simulink model "gui_experiment_supervisor"  (R2024b)
settings: Solver=FixedStepDiscrete  StartTime=0.0  StopTime=inf  FixedStep=Ts  RelTol=1e-3
model workspace (MAT data in the model file):
  Ts = Simulink.Parameter
  Ts.Value = 0.01
  Ts.Complexity = 'real'
  Ts.Dimensions = [1 1]
  Ts.DataType = 'auto'
  Ts.DocUnits = 's'
  board_ID = Simulink.Parameter
  board_ID.Value = 1
  board_ID.Complexity = 'real'
  board_ID.Dimensions = [1 1]
  board_ID.DataType = 'auto'
undefined symbols (not defined in the file): CAN_ANGLE_DEG2ICUB, CAN_ANGLE_ICUB2DEG, canChannel, ControlModes
libraries: canmsglib x12, canlib x4, simulink x1, dspsrcs4 x1, dspsigops x1, dspswit3 x1, sldrtlib x1
settings Model: DataDictionary=amcbldc.sldd  Creator=upattacini  LastModifiedBy=rpumpo
settings SolverCC: AlgebraicLoopSolver=TrustRegion  DecoupledContinuousIntegration=on  MinimalZcImpactIntegration=on
settings OptimizationCC: ReuseModelBlockBuffer=off  SimCompilerOptimization=on
settings DebuggingCC: ParameterPrecisionLossMsg=none  UnconnectedInputMsg=warning  UnconnectedOutputMsg=warning  UnconnectedLineMsg=warning  ArithmeticOperatorsInVariantConditions=warning
settings HardwareCC: ProdBitPerLong=64  ProdHWDeviceType=Intel->x86-64 (Linux 64)
settings ModelReferenceCC: EnableRefExpFcnMdlSchedulingChecks=on
settings SFSimCC: SimUseLocalCustomCode=off  CustomCodeUndefinedFunction=UseInterfaceOnly
settings RTWCC: Description=Simulink Desktop Real-Time  SystemTargetFile=sldrt.tlc  TemplateMakefile=sldrt.tmf  RTWUseLocalCustomCode=off  RTWCompilerOptimization=on  GPUComputeCapability=3.5  DLArmComputeVersion=19.05
settings CodeAppCC: MaxIdLength=95
settings SimulinkDesktopRealTimeCC: TargetLibSuffix=_sldrt.a  TargetPreCompLibLocation=C:\Program Files\MATLAB\R2024b\toolbox\sldrt\lib\win64  ParMdlRefBuildCompliant=on

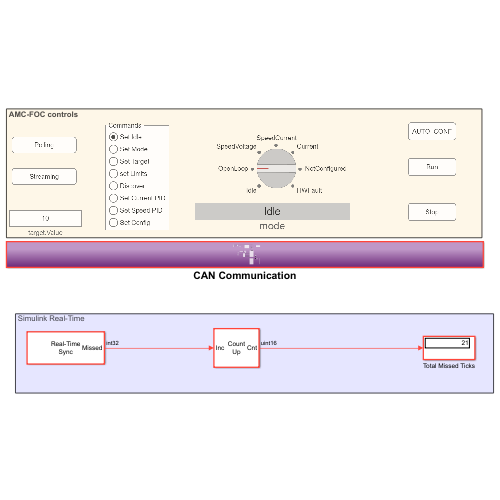
[thumbnail: Simulink's stored preview of the top-level diagram]
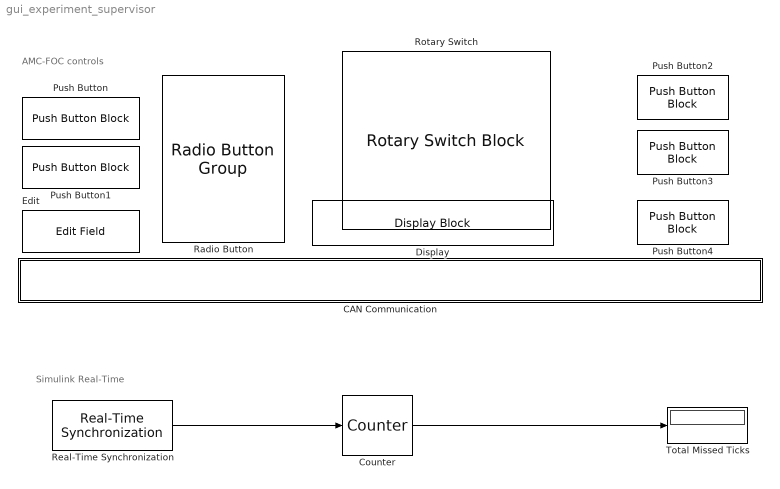
== system gui_experiment_supervisor ==
  note: AMC-FOC controls
  note: Simulink Real-Time
  CAN Communication : Subsystem
  Counter : dspswit3/Counter  Direction=Up  CountEvent=Rising edge  CounterSize=16 bits  MaxCount=10000  InitialCount=0  Output=Count  HitValue=32  ResetInput=off  SamplesPerFrame=1  Ts=1  CntDtype=uint16  HitDtype=Logical
  Display : DisplayBlock  LabelPosition=Bottom  Format=Integer  Transparency=1  FormatString=%s
  Edit : EditField  LabelPosition=Bottom  ShowInitialText=on  Alignment=Center
  Push Button : PushButtonBlock  ButtonText=Polling  OffValue=0.000000
  Push Button1 : PushButtonBlock  ButtonText=Streaming  ButtonType=Latch  OffValue=0.000000
  Push Button2 : PushButtonBlock  ButtonText=AUTO_CONF  OffValue=0.000000
  Push Button3 : PushButtonBlock  ButtonText=Run  OffValue=0.000000
  Push Button4 : PushButtonBlock  ButtonText=Stop  OffValue=0.000000
  Radio Button : RadioButtonGroup  LabelPosition=Hide  SelectedLabel=Set Idle  ButtonGroupName=Commands
      settings: Values={{'Set Idle', 'Set Mode', 'Set Target', 'set Limits', 'Discover', 'Set Current PID', 'Set Speed PID', 'Set Config'}, [1 2 3 4 5 6 7 8]}
  Real-Time Synchronization : sldrtlib/Real-Time Synchronization  SampleTime=Ts  MaxMissedTicks=inf  ShowMissedTicks=on  YieldWhenWaiting=off
  Rotary Switch : RotarySwitchBlock  LabelPosition=Hide  UseEnumeratedDataType=on  EnumeratedDataType=MCControlModes
      settings: Values={{'Idle', 'OpenLoop', 'SpeedVoltage', 'SpeedCurrent', 'Current', 'NotConfigured', 'HWFault'}, [0 80 10 11 6 176 160]}
  Total Missed Ticks : Display
      settings: Decimation=5
  wires:
  Counter/1 -> Total Missed Ticks/1
  Real-Time Synchronization/1 -> Counter/1

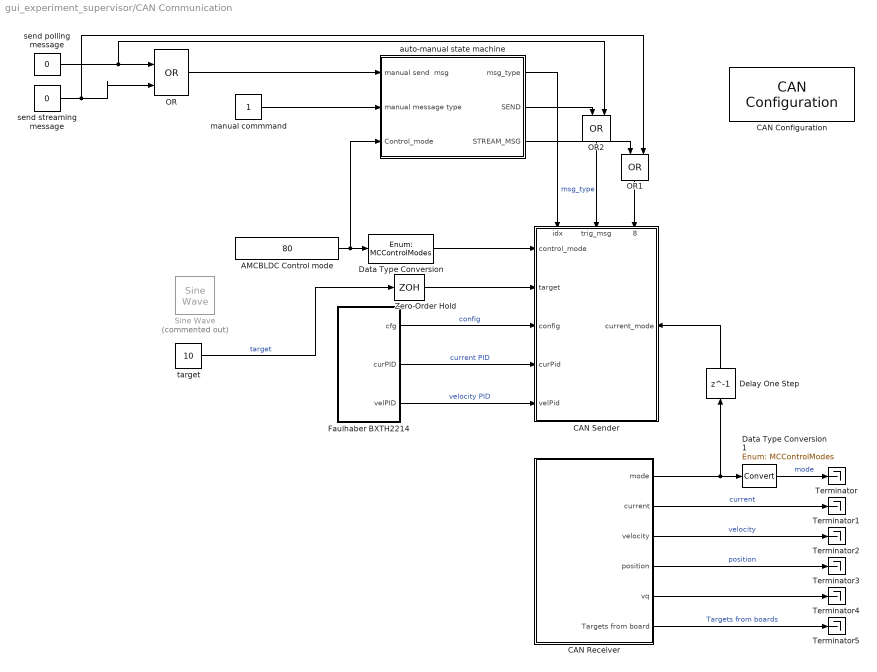
== system gui_experiment_supervisor/CAN Communication ==
  AMCBLDC Control mode : Constant  Value=80  OutDataTypeStr=int16  SampleTime=Ts
  CAN Configuration : canlib/CAN Configuration  BlockHandle=364.0001  Device=Vector VN1610 1 (Channel 1)  DeviceMenu=Vector VN1610 1 (Channel 1)  ObjConstructor=canChannel('Vector', 'VN1610 1', 1)  BusSpeed=1000000  EnableBitParameters=off  SJW=1  TSEG1=4  TSEG2=3  NSamples=1  AckMode=Normal
  CAN Receiver : Subsystem
  CAN Sender : Subsystem
      settings: PortSchema="{\"entries\":[{\"content\":{\"sides\":[{\"content\":{\"connectorIds\":[\"In1\",\"In2\",\"In3\",\"In4\",\"In5\"]},\"type\":\"ConnectorPlacement.EquallySpacedRectSide\",\"uuid\":\"bdd6ce9e-9b65-4aba-9b48-f09f8c1326bb\"},{\"content\":{\"connectorIds\":[\"In9\"],\"side\":\"RIGHT\"},\"type\":\"ConnectorPlacement.EquallySpacedRectSide\",\"uuid\":\"141c9ef5-f742-47fc-b635-015c7474b58f\"},{\"content\":{\"connectorIds\":[\"In6\",\"In7\",\"In8\"],\"side\":\"TOP\"},\"type\":\"ConnectorPlacement.EquallySpacedRectSide\",\"uuid\":\"624889ac-74c5-4b05-9d21-0587daea952f\"}]},\"type\":\"ConnectorPlacement.EquallySpacedConnector\",\"uuid\":\"a748afda-e52d-41b4-a312-ee668058905d\"}],\"packageUris\":[\"http://schema.mathworks.com/mf0/Connector/R2020b\"],\"version\":\"1.0\"}"
  Data Type Conversion : DataTypeConversion  OutDataTypeStr=Enum: MCControlModes  SaturateOnIntegerOverflow=off  RndMeth=Floor
  Data Type Conversion1 : DataTypeConversion  OutDataTypeStr=Enum: MCControlModes  SaturateOnIntegerOverflow=off  RndMeth=Floor
  Delay One Step : Delay  DelayLength=1
  Faulhaber BXTH2214 : Subsystem  TreatAsAtomicUnit=on  SystemSampleTime=Ts
  OR : Logic  Operator=OR  IconShape=distinctive  AllPortsSameDT=off  OutDataTypeStr=boolean
  OR1 : Logic  Operator=OR  IconShape=distinctive  AllPortsSameDT=off  OutDataTypeStr=boolean
  OR2 : Logic  Operator=OR  IconShape=distinctive  AllPortsSameDT=off  OutDataTypeStr=boolean
  Sine Wave : dspsrcs4/Sine Wave  Commented=on  Amplitude=1  Frequency=0.05  Phase=0  SampleMode=Discrete  OutComplex=Real  CompMethod=Trigonometric fcn  TableSize=Speed  SampleTime=1/50  SamplesPerFrame=1  ResetState=Restart at time zero  OutputFrames=off  dataType=double  wordLen=16  udDataType=sfix(16)  fracBitsMode=Best precision  numFracBits=15  OutDataTypeStr=double  LastOutDataTypeStr=double
  Terminator{,1..5} (6 alike) : Terminator
  Zero-Order Hold : ZeroOrderHold  SampleTime=Ts
  auto-manual state machine : Subsystem
  manual commmand : Constant  OutDataTypeStr=int16  SampleTime=Ts
  send polling message : Constant  Value=0  OutDataTypeStr=boolean  SampleTime=Ts
  send streaming message : Constant  Value=0  OutDataTypeStr=boolean  SampleTime=Ts
  target : Constant  Value=10  SampleTime=Ts
  wires:
  Faulhaber BXTH2214/2(curPID) -> CAN Sender/4(curPid)  "current PID"
  OR/1 -> auto-manual state machine/1(manual send  msg)
  Zero-Order Hold/1 -> CAN Sender/2(target)
  AMCBLDC Control mode/1 -> auto-manual state machine/3(Control_mode), Data Type Conversion/1
  CAN Receiver/3(velocity) -> Terminator2/1  "velocity"
  CAN Receiver/6(Targets from board) -> Terminator5/1  "Targets from boards"
  Data Type Conversion/1 -> CAN Sender/1(control_mode)
  Faulhaber BXTH2214/3(velPID) -> CAN Sender/5(velPid)  "velocity PID"
  CAN Receiver/5(vq) -> Terminator4/1
  CAN Receiver/4(position) -> Terminator3/1  "position"
  CAN Receiver/1(mode) -> Data Type Conversion1/1, Delay One Step/1
  manual commmand/1 -> auto-manual state machine/2(manual message type)
  auto-manual state machine/1(msg_type) -> CAN Sender/6(idx)  "msg_type"
  send streaming message/1 -> OR1/2, OR/2
  Data Type Conversion1/1 -> Terminator/1  "mode"
  send polling message/1 -> OR2/2, OR/1
  Delay One Step/1 -> CAN Sender/9(current_mode)
  Faulhaber BXTH2214/1(cfg) -> CAN Sender/3(config)  "config"
  target/1 -> Zero-Order Hold/1  "target"
  CAN Receiver/2(current) -> Terminator1/1  "current"
  auto-manual state machine/3(STREAM_MSG) -> OR1/1
  OR1/1 -> CAN Sender/8(trig_periodic)
  OR2/1 -> CAN Sender/7(trig_msg)
  auto-manual state machine/2(SEND) -> OR2/1

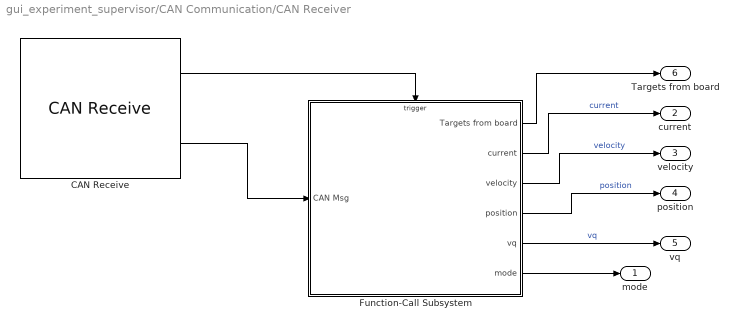
== system gui_experiment_supervisor/CAN Communication/CAN Receiver ==
  CAN Receive : canlib/CAN Receive  BlockHandle=372.0001  Device=Vector VN1610 1 (Channel 1)  DeviceMenu=Vector VN1610 1 (Channel 1)  ObjConstructor=canChannel('Vector', 'VN1610 1', 1)  EnableStandardIDsFilter=off  StdIDsCombo=Allow all  StandardIDs=0  EnableExtendedIDsFilter=off  ExtIDsCombo=Allow all  ExtendedIDs=0  SampleTime=Ts  MsgsPerTimestep=all  InternalFilterUpdateStatus=on  BusOutput=on
  Function-Call Subsystem : Subsystem  TreatAsAtomicUnit=on
  mode : Outport
  current : Outport  Port=2
  velocity : Outport  Port=3
  position : Outport  Port=4
  vq : Outport  Port=5
  Targets from board : Outport  Port=6
  wires:
  CAN Receive/1 -> Function-Call Subsystem/Trigger
  CAN Receive/2 -> Function-Call Subsystem/1(CAN Msg)
  Function-Call Subsystem/2(current) -> current/1  "current"
  Function-Call Subsystem/3(velocity) -> velocity/1  "velocity"
  Function-Call Subsystem/4(position) -> position/1  "position"
  Function-Call Subsystem/5(vq) -> vq/1  "vq"
  Function-Call Subsystem/1(Targets from board) -> Targets from board/1
  Function-Call Subsystem/6(mode) -> mode/1

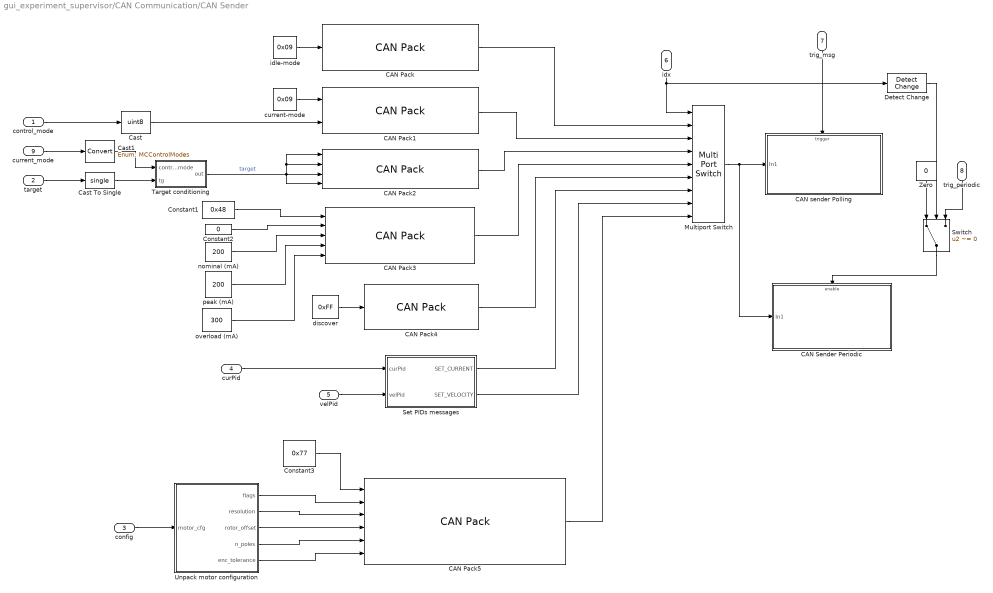
== system gui_experiment_supervisor/CAN Communication/CAN Sender ==
  control_mode : Inport
  target : Inport  Port=2
  config : Inport  Port=3
  curPid : Inport  Port=4
  velPid : Inport  Port=5
  idx : Inport  Port=6
  trig_msg : Inport  Port=7
  trig_periodic : Inport  Port=8
  current_mode : Inport  Port=9
  CAN Pack : canmsglib/CAN Pack  MsgList=(none)  MsgName=CAN Idle  MsgIDType=Standard (11-bit identifier)  MsgIdentifier=board_ID  CANIDInput=off  MsgLength=2  Remote=off  ApplyMinMax=off  BusOutput=on  SignalInfo={ 'Idle', '0', '16', 'LE', 'unsigned', 'Standard', '0', '1', '0', '-Inf', 'Inf' }
      settings: DataFormat=manually specified signals
  CAN Pack1 : canmsglib/CAN Pack  MsgList=(none)  MsgName=SET Control Mode  MsgIDType=Standard (11-bit identifier)  MsgIdentifier=board_ID  CANIDInput=off  MsgLength=2  Remote=off  ApplyMinMax=off  BusOutput=on  SignalInfo={ 'CMD', '0', '8', 'LE', 'unsigned', 'Standard', '0', '1', '0', '-Inf', 'Inf'; 'CTRL', '8', '8', 'LE', 'signed', 'Standard', '0', '1', '0', '-Inf', 'Inf' }
      settings: DataFormat=manually specified signals
  CAN Pack2 : canmsglib/CAN Pack  MsgList=(none)  MsgName=CAN Target  MsgIDType=Standard (11-bit identifier)  MsgIdentifier=0x10F  CANIDInput=off  MsgLength=8  Remote=off  ApplyMinMax=off  BusOutput=on  SignalInfo={ 'Target 1', '0', '16', 'LE', 'signed', 'Standard', '0', '1', '0', '-Inf', 'Inf'; 'Target 2', '16', '16', 'LE', 'signed', 'Standard', '0', '1', '0', '-Inf', 'Inf'; 'Target 3', '32', '16', 'LE', 'signed', 'Standard', '0', '1', '0', '-Inf', 'Inf'; 'Target 4', '48', '16', 'LE', 'signed', 'Standard', '0', '1', '0', '-Inf', 'Inf' }
      settings: DataFormat=manually specified signals
  CAN Pack3 : canmsglib/CAN Pack  MsgList=(none)  MsgName=CAN Limits  MsgIDType=Standard (11-bit identifier)  MsgIdentifier=board_ID  CANIDInput=off  MsgLength=8  Remote=off  ApplyMinMax=off  BusOutput=on  SignalInfo={ 'CMD', '0', '8', 'LE', 'unsigned', 'Standard', '0', '1', '0', '-Inf', 'Inf'; 'X', '8', '8', 'LE', 'unsigned', 'Standard', '0', '1', '0', '-Inf', 'Inf'; 'NOMINAL', '16', '16', 'LE', 'unsigned', 'Standard', '0', '1', '0', '-Inf', 'Inf'; 'PEAK', '32', '16', 'LE', 'unsigned', 'Standard', '0', '1', '0', '-Inf', 'Inf'; 'OVERLOAD', '48', '16', 'LE', 'unsigned', 'Standard', '0', '1', '0', '-Inf', 'Inf' }
      settings: DataFormat=manually specified signals
  CAN Pack4 : canmsglib/CAN Pack  MsgList=(none)  MsgName=DISCOVER  MsgIDType=Standard (11-bit identifier)  MsgIdentifier=0x70F  CANIDInput=off  MsgLength=1  Remote=off  ApplyMinMax=off  BusOutput=on  SignalInfo={}
      settings: DataFormat=raw data
  CAN Pack5 : canmsglib/CAN Pack  MsgList=(none)  MsgName=Set_Motor_Config  MsgIDType=Standard (11-bit identifier)  MsgIdentifier=board_ID  CANIDInput=off  MsgLength=8  Remote=off  ApplyMinMax=off  BusOutput=on  SignalInfo={ 'CMD', '0', '8', 'LE', 'unsigned', 'Standard', '0', '1', '0', '-Inf', 'Inf'; 'FLAGS', '8', '8', 'LE', 'unsigned', 'Standard', '0', '1', '0', '-Inf', 'Inf'; 'RES_ENCODER', '16', '16', 'LE', 'signed', 'Standard', '0', '1', '0', '-Inf', 'Inf'; 'OFFSET_ENCODER', '32', '16', 'LE', 'unsigned', 'Standard', '0', '1', '0', '-Inf', 'Inf'; 'N_POLES', '48', '8', 'LE', 'unsigned', 'Standard', '0', '1', '0', '-Inf', 'Inf'; 'ENCODER_TOLERANCE', '56', '8', 'LE', 'unsigned', 'Standard', '0', '1', '0', '-Inf', 'Inf' }
      settings: DataFormat=manually specified signals
  CAN Sender Periodic : Subsystem  TreatAsAtomicUnit=on
  CAN sender Polling : Subsystem
  Cast : DataTypeConversion  OutDataTypeStr=uint8  SaturateOnIntegerOverflow=off  RndMeth=Floor
  Cast To Single : DataTypeConversion  OutDataTypeStr=single  SaturateOnIntegerOverflow=off  RndMeth=Floor
  Cast1 : DataTypeConversion  OutDataTypeStr=Enum: MCControlModes  SaturateOnIntegerOverflow=off  RndMeth=Floor
  Constant1 : Constant  Value=0x48  OutDataTypeStr=Inherit: Inherit via back propagation
  Constant2 : Constant  Value=0  OutDataTypeStr=Inherit: Inherit via back propagation
  Constant3 : Constant  Value=0x77  OutDataTypeStr=Inherit: Inherit via back propagation
  Detect Change : simulink/Logic and Bit Operations/Detect Change  vinit=0  OutDataTypeStr=boolean
  Multiport Switch : MultiPortSwitch  Inputs=8  DiagnosticForDefault=Warning  SaturateOnIntegerOverflow=off  InputSameDT=off
  Set PIDs messages : Subsystem
  Switch : Switch  Criteria=u2 ~= 0  SaturateOnIntegerOverflow=off  InputSameDT=off
  Target conditioning : Subsystem
  Unpack motor configuration : MATLAB Function  TreatAsAtomicUnit=on
  Zero : Constant  Value=0  OutDataTypeStr=Inherit: Inherit via back propagation
  current-mode : Constant  Value=0x09  OutDataTypeStr=Inherit: Inherit via back propagation
  discover : Constant  Value=0xFF
  idle-mode : Constant  Value=0x09  OutDataTypeStr=Inherit: Inherit via back propagation
  nominal (mA) : Constant  Value=200  OutDataTypeStr=Inherit: Inherit via back propagation
  overload (mA) : Constant  Value=300  OutDataTypeStr=Inherit: Inherit via back propagation
  peak (mA) : Constant  Value=200  OutDataTypeStr=Inherit: Inherit via back propagation
  wires:
  CAN Pack/1 -> Multiport Switch/2
  CAN Pack1/1 -> Multiport Switch/3
  CAN Pack2/1 -> Multiport Switch/4
  idx/1 -> Multiport Switch/1, Detect Change/1
  idle-mode/1 -> CAN Pack/1
  current-mode/1 -> CAN Pack1/1
  Constant1/1 -> CAN Pack3/1
  CAN Pack3/1 -> Multiport Switch/5
  discover/1 -> CAN Pack4/1
  CAN Pack4/1 -> Multiport Switch/6
  trig_msg/1 -> CAN sender Polling/Trigger
  Constant2/1 -> CAN Pack3/2
  nominal (mA)/1 -> CAN Pack3/3
  peak (mA)/1 -> CAN Pack3/4
  overload (mA)/1 -> CAN Pack3/5
  trig_periodic/1 -> Switch/3
  Multiport Switch/1 -> CAN Sender Periodic/1(In1), CAN sender Polling/1(In1)
  control_mode/1 -> Cast/1
  Constant3/1 -> CAN Pack5/1
  Set PIDs messages/2(SET_VELOCITY) -> Multiport Switch/8
  Set PIDs messages/1(SET_CURRENT) -> Multiport Switch/7
  velPid/1 -> Set PIDs messages/2(velPid)
  CAN Pack5/1 -> Multiport Switch/9
  config/1 -> Unpack motor configuration/1(motor_cfg)
  curPid/1 -> Set PIDs messages/1(curPid)
  Unpack motor configuration/1(flags) -> CAN Pack5/2
  Unpack motor configuration/2(resolution) -> CAN Pack5/3
  Unpack motor configuration/3(rotor_offset) -> CAN Pack5/4
  Unpack motor configuration/4(n_poles) -> CAN Pack5/5
  Unpack motor configuration/5(enc_tolerance) -> CAN Pack5/6
  target/1 -> Cast To Single/1
  Target conditioning/1(out) -> CAN Pack2/4, CAN Pack2/1, CAN Pack2/2, CAN Pack2/3  "target"
  Cast/1 -> CAN Pack1/2
  Cast1/1 -> Target conditioning/1(control_mode)
  current_mode/1 -> Cast1/1
  Detect Change/1 -> Switch/2
  Zero/1 -> Switch/1
  Switch/1 -> CAN Sender Periodic/Enable
  Cast To Single/1 -> Target conditioning/2(tg)

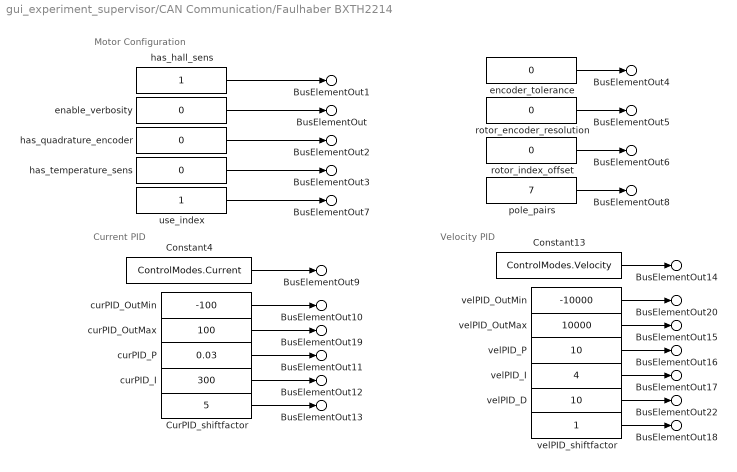
== system gui_experiment_supervisor/CAN Communication/Faulhaber BXTH2214 ==
  note: Motor Configuration
  note: Current PID
  note: Velocity PID
  Constant13 : Constant  Value=ControlModes.Velocity  OutDataTypeStr=Inherit: Inherit via back propagation
  Constant4 : Constant  Value=ControlModes.Current  OutDataTypeStr=Inherit: Inherit via back propagation
  CurPID_shiftfactor : Constant  Value=5  OutDataTypeStr=Inherit: Inherit via back propagation
  curPID_I : Constant  Value=300  OutDataTypeStr=Inherit: Inherit via back propagation
  curPID_OutMax : Constant  Value=100  OutDataTypeStr=Inherit: Inherit via back propagation
  curPID_OutMin : Constant  Value=-100  OutDataTypeStr=Inherit: Inherit via back propagation
  curPID_P : Constant  Value=0.03  OutDataTypeStr=Inherit: Inherit via back propagation
  enable_verbosity : Constant  Value=0  OutDataTypeStr=boolean
  encoder_tolerance : Constant  Value=0  OutDataTypeStr=Inherit: Inherit via back propagation
  has_hall_sens : Constant  OutDataTypeStr=boolean
  has_quadrature_encoder : Constant  Value=0  OutDataTypeStr=boolean
  has_temperature_sens : Constant  Value=0  OutDataTypeStr=boolean
  pole_pairs : Constant  Value=7  OutDataTypeStr=Inherit: Inherit via back propagation
  rotor_encoder_resolution : Constant  Value=0  OutDataTypeStr=Inherit: Inherit via back propagation
  rotor_index_offset : Constant  Value=0  OutDataTypeStr=Inherit: Inherit via back propagation
  use_index : Constant  OutDataTypeStr=boolean
  velPID_D : Constant  Value=10  OutDataTypeStr=Inherit: Inherit via back propagation
  velPID_I : Constant  Value=4  OutDataTypeStr=Inherit: Inherit via back propagation
  velPID_OutMax : Constant  Value=10000  OutDataTypeStr=Inherit: Inherit via back propagation
  "velPID_OutMin " : Constant  Value=-10000  OutDataTypeStr=Inherit: Inherit via back propagation
  velPID_P : Constant  Value=10  OutDataTypeStr=Inherit: Inherit via back propagation
  velPID_shiftfactor : Constant  OutDataTypeStr=Inherit: Inherit via back propagation
  BusElementOut : Outport  PortName=cfg  Element=enable_verbosity
  BusElementOut1 : Outport  PortName=cfg  Element=has_hall_sens
  BusElementOut2 : Outport  PortName=cfg  Element=has_quadrature_encoder
  BusElementOut3 : Outport  PortName=cfg  Element=has_temperature_sens
  BusElementOut4 : Outport  PortName=cfg  Element=encoder_tolerance
  BusElementOut8 : Outport  PortName=cfg  Element=pole_pairs
  BusElementOut5 : Outport  PortName=cfg  Element=rotor_encoder_resolution
  BusElementOut6 : Outport  PortName=cfg  Element=rotor_index_offset
  BusElementOut7 : Outport  PortName=cfg  Element=use_index
  BusElementOut9 : Outport  Port=2  PortName=curPID  Element=type
  BusElementOut19 : Outport  Port=2  PortName=curPID  Element=OutMax
  BusElementOut10 : Outport  Port=2  PortName=curPID  Element=OutMin
  BusElementOut11 : Outport  Port=2  PortName=curPID  Element=P
  BusElementOut12 : Outport  Port=2  PortName=curPID  Element=I
  BusElementOut13 : Outport  Port=2  PortName=curPID  Element=shift_factor
  BusElementOut14 : Outport  Port=3  PortName=velPID  Element=type
  BusElementOut15 : Outport  Port=3  PortName=velPID  Element=OutMax
  BusElementOut20 : Outport  Port=3  PortName=velPID  Element=OutMin
  BusElementOut16 : Outport  Port=3  PortName=velPID  Element=P
  BusElementOut17 : Outport  Port=3  PortName=velPID  Element=I
  BusElementOut22 : Outport  Port=3  PortName=velPID  Element=D
  BusElementOut18 : Outport  Port=3  PortName=velPID  Element=shift_factor
  wires:
  encoder_tolerance/1 -> BusElementOut4/1
  pole_pairs/1 -> BusElementOut8/1
  Constant4/1 -> BusElementOut9/1
  curPID_OutMin/1 -> BusElementOut10/1
  curPID_P/1 -> BusElementOut11/1
  curPID_OutMax/1 -> BusElementOut19/1
  curPID_I/1 -> BusElementOut12/1
  CurPID_shiftfactor/1 -> BusElementOut13/1
  velPID_I/1 -> BusElementOut17/1
  velPID_shiftfactor/1 -> BusElementOut18/1
  velPID_P/1 -> BusElementOut16/1
  Constant13/1 -> BusElementOut14/1
  rotor_encoder_resolution/1 -> BusElementOut5/1
  rotor_index_offset/1 -> BusElementOut6/1
  "velPID_OutMin "/1 -> BusElementOut20/1
  velPID_OutMax/1 -> BusElementOut15/1
  velPID_D/1 -> BusElementOut22/1
  enable_verbosity/1 -> BusElementOut/1
  has_quadrature_encoder/1 -> BusElementOut2/1
  has_temperature_sens/1 -> BusElementOut3/1
  use_index/1 -> BusElementOut7/1
  has_hall_sens/1 -> BusElementOut1/1

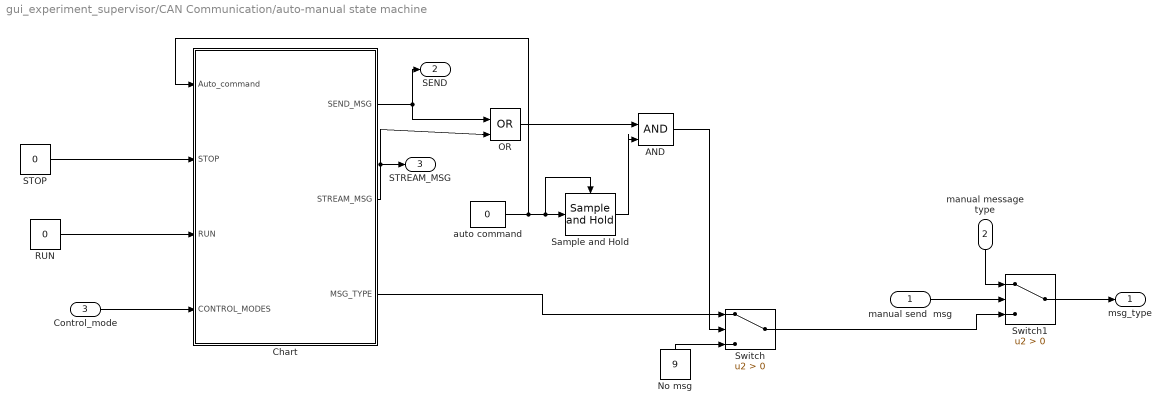
== system gui_experiment_supervisor/CAN Communication/auto-manual state machine ==
  manual send  msg : Inport
  manual message type : Inport  Port=2
  Control_mode : Inport  Port=3
  AND : Logic  IconShape=distinctive  AllPortsSameDT=off  OutDataTypeStr=boolean
  Chart : Stateflow chart  TreatAsAtomicUnit=on
      settings: PortSchema="{\"entries\":[{\"content\":{\"sides\":[{\"content\":{\"connectorIds\":[\"In1\",\"In3\",\"In2\",\"In4\"]},\"type\":\"ConnectorPlacement.EquallySpacedRectSide\",\"uuid\":\"3f3ecf7a-eca8-49e2-a594-4c8df01bcae2\"},{\"content\":{\"connectorIds\":[\"Out2\",\"Out3\",\"Out1\"],\"side\":\"RIGHT\"},\"type\":\"ConnectorPlacement.EquallySpacedRectSide\",\"uuid\":\"2e405059-6050-4daf-b42b-e1c8d6f3a572\"},{\"content\":{\"side\":\"TOP\"},\"type\":\"ConnectorPlacement.EquallySpacedRectSide\",\"uuid\":\"8705f6e5-e301-4990-b24d-44270950b42f\"}]},\"type\":\"ConnectorPlacement.EquallySpacedConnector\",\"uuid\":\"46b9b7aa-14e0-48f8-b8fe-455c7835f2bb\"}],\"packageUris\":[\"http://schema.mathworks.com/mf0/Connector/R2020b\"],\"version\":\"1.0\"}"
  No msg : Constant  Value=9  OutDataTypeStr=Inherit: Inherit via back propagation
  OR : Logic  Operator=OR  IconShape=distinctive  AllPortsSameDT=off  OutDataTypeStr=boolean
  RUN : Constant  Value=0
  STOP : Constant  Value=0
  Sample and Hold : dspsigops/Sample and Hold  trig=Rising edge  initCond=0  latchinput=off
  Switch : Switch  Criteria=u2 > Threshold  SaturateOnIntegerOverflow=off  InputSameDT=off
  Switch1 : Switch  Criteria=u2 > Threshold  SaturateOnIntegerOverflow=off  InputSameDT=off
  auto command : Constant  Value=0
  msg_type : Outport
  SEND : Outport  Port=2
  STREAM_MSG : Outport  Port=3
  wires:
  manual send  msg/1 -> Switch1/2
  manual message type/1 -> Switch1/1
  Switch1/1 -> msg_type/1
  Control_mode/1 -> Chart/4(CONTROL_MODES)
  Chart/2(SEND_MSG) -> SEND/1, OR/1
  auto command/1 -> Chart/1(Auto_command), Sample and Hold/1, Sample and Hold/Trigger
  Sample and Hold/1 -> AND/2
  RUN/1 -> Chart/2(RUN)
  STOP/1 -> Chart/3(STOP)
  No msg/1 -> Switch/3
  AND/1 -> Switch/2
  Chart/1(MSG_TYPE) -> Switch/1
  Switch/1 -> Switch1/3
  Chart/3(STREAM_MSG) -> OR/2, STREAM_MSG/1
  OR/1 -> AND/1

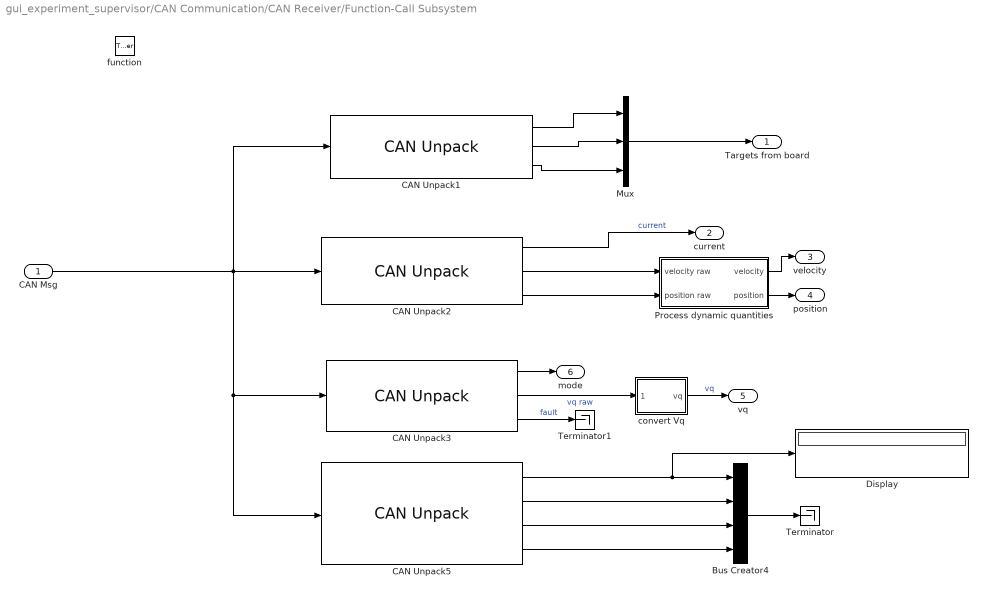
== system gui_experiment_supervisor/CAN Communication/CAN Receiver/Function-Call Subsystem ==
  CAN Msg : Inport
  function : TriggerPort  TriggerType=function-call  VariantControl=(inherit)
  Bus Creator4 : BusCreator  Inputs=4
  CAN Unpack1 : canmsglib/CAN Unpack  MsgList=(none)  MsgName=TARGETS  MsgIDType=Standard (11-bit identifier)  MsgIdentifier=0x10F  MsgLength=8  SignalInfo={ 'Target1', '0', '16', 'LE', 'signed', 'Standard', '0', '1', '0', '-Inf', 'Inf'; 'Target2', '16', '16', 'LE', 'signed', 'Standard', '0', '1', '0', '-Inf', 'Inf'; 'Target3', '32', '16', 'LE', 'signed', 'Standard', '0', '1', '0', '-Inf', 'Inf' }  IDPort=off  TimestampPort=off  ErrorPort=off  RemotePort=off  LengthPort=off  StatusPort=off  ApplyMinMax=off
  CAN Unpack2 : canmsglib/CAN Unpack  MsgList=(none)  MsgName=FOC  MsgIDType=Standard (11-bit identifier)  MsgIdentifier=0x110  MsgLength=8  SignalInfo={ 'current', '0', '16', 'LE', 'signed', 'Standard', '0', '1', '0', '-Inf', 'Inf'; 'velocity', '16', '16', 'LE', 'signed', 'Standard', '0', '1', '0', '-Inf', 'Inf'; 'position', '32', '32', 'LE', 'signed', 'Standard', '0', '1', '0', '-Inf', 'Inf' }  IDPort=off  TimestampPort=off  ErrorPort=off  RemotePort=off  LengthPort=off  StatusPort=off  ApplyMinMax=off
  CAN Unpack3 : canmsglib/CAN Unpack  MsgList=(none)  MsgName=STATUS  MsgIDType=Standard (11-bit identifier)  MsgIdentifier=0x113  MsgLength=8  SignalInfo={ 'mode', '0', '8', 'LE', 'unsigned', 'Standard', '0', '1', '0', '-Inf', 'Inf'; 'pwm', '16', '16', 'LE', 'unsigned', 'Standard', '0', '1', '0', '-Inf', 'Inf'; 'fault', '32', '8', 'LE', 'unsigned', 'Standard', '0', '1', '0', '-Inf', 'Inf' }  IDPort=off  TimestampPort=off  ErrorPort=off  RemotePort=off  LengthPort=off  StatusPort=off  ApplyMinMax=off
  CAN Unpack5 : canmsglib/CAN Unpack  MsgList=(none)  MsgName=DISCOVER  MsgIDType=Standard (11-bit identifier)  MsgIdentifier=0x710  MsgLength=5  SignalInfo={}  IDPort=on  TimestampPort=on  ErrorPort=off  RemotePort=off  LengthPort=on  StatusPort=off  ApplyMinMax=off
      settings: DataFormat=raw data
  Display : Display
      settings: Format=hex (Stored Integer)
  Mux : Mux  Inputs=3
  Process dynamic quantities : Subsystem
  Terminator : Terminator
  Terminator1 : Terminator
  convert Vq : Subsystem
  Targets from board : Outport
  current : Outport  Port=2  Unit=mA
  velocity : Outport  Port=3  Unit=deg/s
  position : Outport  Port=4  Unit=deg
  vq : Outport  Port=5  Unit=%  PortDimensions=1
  mode : Outport  Port=6  OutDataTypeStr=uint8
  wires:
  CAN Unpack5/4 -> Bus Creator4/4
  CAN Unpack5/3 -> Bus Creator4/3
  CAN Unpack5/2 -> Bus Creator4/2
  CAN Unpack5/1 -> Display/1, Bus Creator4/1
  Bus Creator4/1 -> Terminator/1
  CAN Unpack1/1 -> Mux/1
  CAN Unpack1/2 -> Mux/2
  CAN Unpack1/3 -> Mux/3
  Mux/1 -> Targets from board/1
  CAN Unpack2/2 -> Process dynamic quantities/1(velocity raw)
  CAN Unpack2/1 -> current/1  "current"
  Process dynamic quantities/2(position) -> position/1
  Process dynamic quantities/1(velocity) -> velocity/1
  CAN Unpack2/3 -> Process dynamic quantities/2(position raw)
  CAN Unpack3/2 -> convert Vq/1(vq raw)  "vq raw"
  CAN Unpack3/1 -> mode/1
  convert Vq/1(vq) -> vq/1  "vq"
  CAN Msg/1 -> CAN Unpack1/1, CAN Unpack2/1, CAN Unpack5/1, CAN Unpack3/1
  CAN Unpack3/3 -> Terminator1/1  "fault"

== system gui_experiment_supervisor/CAN Communication/CAN Sender/CAN Sender Periodic ==
  In1 : Inport
  Enable : EnablePort
  CAN Transmit : canlib/CAN Transmit  BlockHandle=607.0004  Device=Vector VN1610 1 (Channel 1)  DeviceMenu=Vector VN1610 1 (Channel 1)  ObjConstructor=canChannel('Vector', 'VN1610 1', 1)  EnableEventTransmit=off  EnablePeriodicTransmit=on  MessagePeriod=Ts
  wires:
  In1/1 -> CAN Transmit/1

== system gui_experiment_supervisor/CAN Communication/CAN Sender/CAN sender Polling ==
  In1 : Inport
  Trigger : TriggerPort  VariantControl=(inherit)  PortDimensions=1
  CAN Transmit : canlib/CAN Transmit  BlockHandle=616.0004  Device=Vector VN1610 1 (Channel 1)  DeviceMenu=Vector VN1610 1 (Channel 1)  ObjConstructor=canChannel('Vector', 'VN1610 1', 1)  EnableEventTransmit=off  EnablePeriodicTransmit=off  MessagePeriod=1.000
  wires:
  In1/1 -> CAN Transmit/1

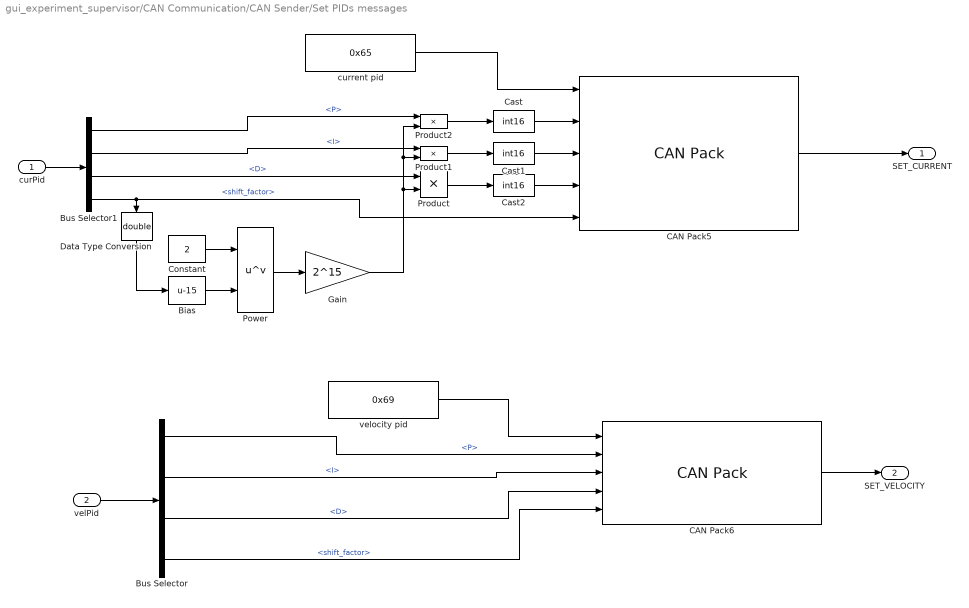
== system gui_experiment_supervisor/CAN Communication/CAN Sender/Set PIDs messages ==
  curPid : Inport
  velPid : Inport  Port=2
  Bias : Bias  Bias=-15  SaturateOnIntegerOverflow=off
  Bus Selector : BusSelector  OutputSignals=P,I,D,shift_factor
  Bus Selector1 : BusSelector  OutputSignals=P,I,D,shift_factor
  CAN Pack5 : canmsglib/CAN Pack  MsgList=(none)  MsgName=SET_CURRENT_PID  MsgIDType=Standard (11-bit identifier)  MsgIdentifier=board_ID  CANIDInput=off  MsgLength=8  Remote=off  ApplyMinMax=off  BusOutput=on  SignalInfo={ 'CMD', '0', '8', 'LE', 'unsigned', 'Standard', '0', '1', '0', '-Inf', 'Inf'; 'Kp', '8', '16', 'LE', 'signed', 'Standard', '0', '1', '0', '-Inf', 'Inf'; 'Ki', '24', '16', 'LE', 'signed', 'Standard', '0', '1', '0', '-Inf', 'Inf'; 'Kd', '40', '16', 'LE', 'signed', 'Standard', '0', '1', '0', '-Inf', 'Inf'; 'shift', '56', '8', 'LE', 'unsigned', 'Standard', '0', '1', '0', '-Inf', 'Inf' }
      settings: DataFormat=manually specified signals
  CAN Pack6 : canmsglib/CAN Pack  MsgList=(none)  MsgName=SET_VELOCITY_PID  MsgIDType=Standard (11-bit identifier)  MsgIdentifier=board_ID  CANIDInput=off  MsgLength=8  Remote=off  ApplyMinMax=off  BusOutput=on  SignalInfo={ 'CMD', '0', '8', 'LE', 'unsigned', 'Standard', '0', '1', '0', '-Inf', 'Inf'; 'Kp', '8', '16', 'LE', 'signed', 'Standard', '0', '1', '0', '-Inf', 'Inf'; 'Ki', '24', '16', 'LE', 'signed', 'Standard', '0', '1', '0', '-Inf', 'Inf'; 'Kd', '40', '16', 'LE', 'signed', 'Standard', '0', '1', '0', '-Inf', 'Inf'; 'shift', '56', '8', 'LE', 'unsigned', 'Standard', '0', '1', '0', '-Inf', 'Inf' }
      settings: DataFormat=manually specified signals
  Cast : DataTypeConversion  OutDataTypeStr=int16  SaturateOnIntegerOverflow=off  RndMeth=Floor
  Cast1 : DataTypeConversion  OutDataTypeStr=int16  SaturateOnIntegerOverflow=off  RndMeth=Floor
  Cast2 : DataTypeConversion  OutDataTypeStr=int16  SaturateOnIntegerOverflow=off  RndMeth=Floor
  Constant : Constant  Value=2
  Data Type Conversion : DataTypeConversion  OutDataTypeStr=double  SaturateOnIntegerOverflow=off  RndMeth=Floor
  Gain : Gain  Gain=2^15  OutDataTypeStr=single
  Power : Math  Operator=pow
  Product : Product
  Product1 : Product
  Product2 : Product
  current pid : Constant  Value=0x65  OutDataTypeStr=int16
  velocity pid : Constant  Value=0x69  OutDataTypeStr=int16
  SET_CURRENT : Outport
  SET_VELOCITY : Outport  Port=2
  wires:
  Bus Selector/4 -> CAN Pack6/5  "<shift_factor>"
  Bus Selector/1 -> CAN Pack6/2  "<P>"
  Bus Selector1/4 -> CAN Pack5/5, Data Type Conversion/1  "<shift_factor>"
  Bus Selector1/1 -> Product2/1  "<P>"
  Bus Selector/3 -> CAN Pack6/4  "<D>"
  Bus Selector/2 -> CAN Pack6/3  "<I>"
  Bus Selector1/2 -> Product1/1  "<I>"
  current pid/1 -> CAN Pack5/1
  velocity pid/1 -> CAN Pack6/1
  CAN Pack5/1 -> SET_CURRENT/1
  CAN Pack6/1 -> SET_VELOCITY/1
  velPid/1 -> Bus Selector/1
  curPid/1 -> Bus Selector1/1
  Bus Selector1/3 -> Product/1  "<D>"
  Power/1 -> Gain/1
  Gain/1 -> Product2/2, Product1/2, Product/2
  Product/1 -> Cast2/1
  Product1/1 -> Cast1/1
  Product2/1 -> Cast/1
  Cast/1 -> CAN Pack5/2
  Cast1/1 -> CAN Pack5/3
  Cast2/1 -> CAN Pack5/4
  Constant/1 -> Power/1
  Bias/1 -> Power/2
  Data Type Conversion/1 -> Bias/1

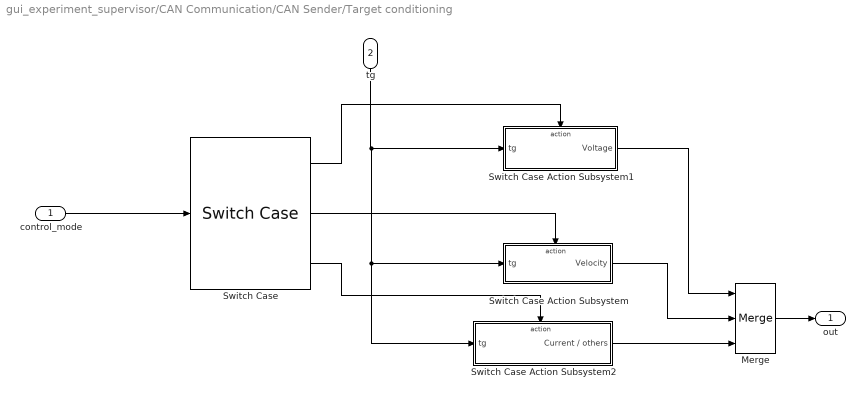
== system gui_experiment_supervisor/CAN Communication/CAN Sender/Target conditioning ==
  control_mode : Inport
  tg : Inport  Port=2
  Merge : Merge  Inputs=3
  Switch Case : SwitchCase  CaseConditions={MCControlModes.OpenLoop, MCControlModes.SpeedVoltage}
  Switch Case Action Subsystem : Subsystem  TreatAsAtomicUnit=on
  Switch Case Action Subsystem1 : Subsystem  TreatAsAtomicUnit=on
  Switch Case Action Subsystem2 : Subsystem  TreatAsAtomicUnit=on
  out : Outport
  wires:
  tg/1 -> Switch Case Action Subsystem2/1(tg), Switch Case Action Subsystem/1(tg), Switch Case Action Subsystem1/1(tg)
  Switch Case/1 -> Switch Case Action Subsystem1/Action
  Switch Case/2 -> Switch Case Action Subsystem/Action
  Switch Case/3 -> Switch Case Action Subsystem2/Action
  Merge/1 -> out/1
  control_mode/1 -> Switch Case/1
  Switch Case Action Subsystem1/1(Voltage) -> Merge/1
  Switch Case Action Subsystem/1(Velocity) -> Merge/2
  Switch Case Action Subsystem2/1(Current / others) -> Merge/3

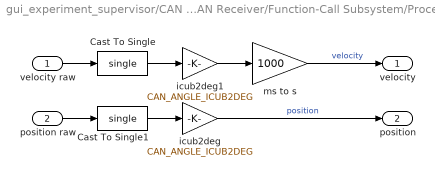
== system gui_experiment_supervisor/CAN Communication/CAN Receiver/Function-Call Subsystem/Process dynamic quantities ==
  velocity raw : Inport
  position raw : Inport  Port=2
  Cast To Single : DataTypeConversion  OutDataTypeStr=single  SaturateOnIntegerOverflow=off  RndMeth=Floor
  Cast To Single1 : DataTypeConversion  OutDataTypeStr=single  SaturateOnIntegerOverflow=off  RndMeth=Floor
  icub2deg : Gain  Gain=CAN_ANGLE_ICUB2DEG
  icub2deg1 : Gain  Gain=CAN_ANGLE_ICUB2DEG
  ms to s : Gain  Gain=1000
  velocity : Outport
  position : Outport  Port=2
  wires:
  Cast To Single1/1 -> icub2deg/1
  icub2deg1/1 -> ms to s/1
  Cast To Single/1 -> icub2deg1/1
  icub2deg/1 -> position/1  "position"
  velocity raw/1 -> Cast To Single/1
  position raw/1 -> Cast To Single1/1
  ms to s/1 -> velocity/1  "velocity"

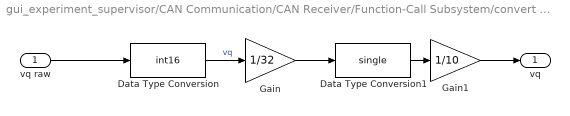
== system gui_experiment_supervisor/CAN Communication/CAN Receiver/Function-Call Subsystem/convert Vq ==
  vq raw : Inport
  Data Type Conversion : DataTypeConversion  OutDataTypeStr=int16  SaturateOnIntegerOverflow=off  RndMeth=Floor
  Data Type Conversion1 : DataTypeConversion  OutDataTypeStr=single  SaturateOnIntegerOverflow=off  RndMeth=Floor
  Gain : Gain  Gain=1/32
  Gain1 : Gain  Gain=1/10
  vq : Outport
  wires:
  vq raw/1 -> Data Type Conversion/1
  Gain/1 -> Data Type Conversion1/1
  Data Type Conversion/1 -> Gain/1  "vq"
  Data Type Conversion1/1 -> Gain1/1
  Gain1/1 -> vq/1

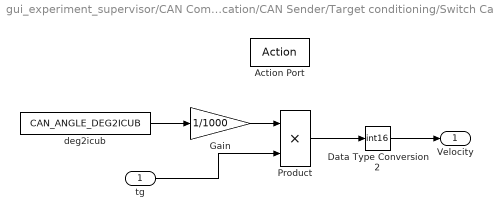
== system gui_experiment_supervisor/CAN Communication/CAN Sender/Target conditioning/Switch Case Action Subsystem ==
  tg : Inport
  Action Port : ActionPort  ActionPortLabel=case [ SpeedVoltage ]:
  Data Type Conversion2 : DataTypeConversion  OutDataTypeStr=int16  SaturateOnIntegerOverflow=off  RndMeth=Floor
  Gain : Gain  Gain=1/1000
  Product : Product
  deg2icub : Constant  Value=CAN_ANGLE_DEG2ICUB  OutDataTypeStr=single
  Velocity : Outport
  wires:
  tg/1 -> Product/2
  Gain/1 -> Product/1
  deg2icub/1 -> Gain/1
  Product/1 -> Data Type Conversion2/1
  Data Type Conversion2/1 -> Velocity/1

== system gui_experiment_supervisor/CAN Communication/CAN Sender/Target conditioning/Switch Case Action Subsystem1 ==
  tg : Inport
  Action Port : ActionPort  ActionPortLabel=case [ OpenLoop ]:
  Data Type Conversion : DataTypeConversion  OutDataTypeStr=int16  SaturateOnIntegerOverflow=off  RndMeth=Floor
  Gain : Gain  Gain=32
  Gain1 : Gain  Gain=10
  Voltage : Outport
  wires:
  Gain1/1 -> Gain/1
  tg/1 -> Gain1/1
  Data Type Conversion/1 -> Voltage/1
  Gain/1 -> Data Type Conversion/1

== system gui_experiment_supervisor/CAN Communication/CAN Sender/Target conditioning/Switch Case Action Subsystem2 ==
  tg : Inport
  Action Port : ActionPort  ActionPortLabel=default:
  Data Type Conversion3 : DataTypeConversion  OutDataTypeStr=int16  SaturateOnIntegerOverflow=off  RndMeth=Floor
  Current / others : Outport
  wires:
  tg/1 -> Data Type Conversion3/1
  Data Type Conversion3/1 -> Current / others/1

== stateflow chart gui_experiment_supervisor/CAN Communication/auto-manual state machine/Chart ==
  state NotConfigured
    entry:
    SEND_MSG = 1;
    MSG_TYPE = 4;
    during:
    SEND_MSG = 0;
  state Set_Limits
    entry:
    SEND_MSG = 1;
    MSG_TYPE = 4;
    exit:
    SEND_MSG = 0;
  state MotorConfig
    entry:
    SEND_MSG = 1;
    MSG_TYPE = 8;
    exit:
    SEND_MSG = 0;
  state Set_Current_PID
    entry:
    SEND_MSG = 1;
    MSG_TYPE = 6;
    exit:
    SEND_MSG = 0;
  state Set_Speed_PID
    entry:
    SEND_MSG = 1;
    MSG_TYPE = 7;
    exit:
    SEND_MSG = 0;
  state Idle
    entry:
    SEND_MSG = 1;
    MSG_TYPE = 1;
    Local_stop = 0;
    during :
    SEND_MSG = 0;
  state Set_Target
    entry:
    STREAM_MSG = 1;
    MSG_TYPE = 3;
    during:
    if (STOP == 1)
    Local_stop = 1;
    end
    exit:
    STREAM_MSG =0;
  state Set_Mode
    entry:
    SEND_MSG = 1;
    MSG_TYPE = 2;
    exit :
    Memory_cntrl = CONTROL_MODES;
    SEND_MSG = 0;
  (default) -> NotConfigured
  NotConfigured -> Set_Limits : [Auto_command~=0]
  Idle -> Set_Limits [order 1] : [Auto_command~=0]
  Set_Limits -> MotorConfig : [after(1,sec)]
  MotorConfig -> Set_Current_PID : [after(1,sec)]
  Set_Current_PID -> Set_Speed_PID : [after(1,sec)]
  Set_Speed_PID -> Idle : [after(1,sec)]
  Set_Target -> Idle [order 1] : [Local_stop ==1]
  Set_Target -> Set_Mode [order 2] : [CONTROL_MODES~= Memory_cntrl]
  Idle -> Set_Mode [order 2] : [RUN ~= 0 ]
  Set_Mode -> Set_Target : [after(1,sec) && CONTROL_MODES~=0 && CONTROL_MODES ~=176 && CONTROL_MODES ~=160 ]
  data: Auto_command input; RUN input; STOP input; MSG_TYPE output uint8 =uint8(1); CONTROL_MODES input; SEND_MSG output uint8 =uint8(0); Memory_cntrl local; Local_stop local; STREAM_MSG output

== matlab function gui_experiment_supervisor/CAN Communication/CAN Sender/Unpack motor configuration ==
  data: flags output; resolution output; rotor_offset output; n_poles output; motor_cfg input; enc_tolerance output
function [flags, resolution,rotor_offset, n_poles, enc_tolerance] = unpack_cfg(motor_cfg)

    flags = uint8(motor_cfg.has_quadrature_encoder); 
    flags = bitor(flags, bitshift(uint8(motor_cfg.has_hall_sens), 1));
    resolution = motor_cfg.rotor_encoder_resolution;
    rotor_offset = motor_cfg.rotor_index_offset;
    n_poles = motor_cfg.pole_pairs * 2;
    enc_tolerance = motor_cfg.encoder_tolerance;

end
